simulink model "SS5"  (R2020a)
settings: Solver=VariableStepAuto  StartTime=0.0  StopTime=10.0  RelTol=1e-3
settings Model: Creator=Asus  LastModifiedBy=Asus

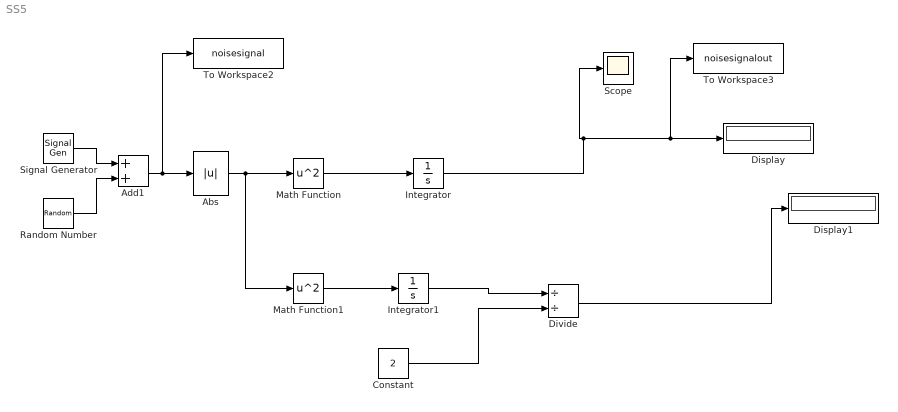
== system SS5 ==
  Abs : Abs
  Add1 : Sum
  Constant : Constant  Value=2
  Display : Display
  Display1 : Display
  Divide : Product  Inputs=//
  Integrator : Integrator  LimitOutput=on
  Integrator1 : Integrator  LimitOutput=on
  Math Function : Math  Operator=square  SaturateOnIntegerOverflow=on
  Math Function1 : Math  Operator=square  SaturateOnIntegerOverflow=on
  Random Number : RandomNumber  SampleTime=0.1
  Scope : Scope
  Signal Generator : SignalGenerator  Units=rad/sec
  To Workspace2 : ToWorkspace  VariableName=noisesignal  SaveFormat=Timeseries  SampleTime=-1
  To Workspace3 : ToWorkspace  VariableName=noisesignalout  SaveFormat=Timeseries  SampleTime=-1
  wires:
  Abs/1 -> Math Function1/1, Math Function/1
  Integrator1/1 -> Divide/1
  Divide/1 -> Display1/1
  Math Function/1 -> Integrator/1
  Math Function1/1 -> Integrator1/1
  Constant/1 -> Divide/2
  Integrator/1 -> To Workspace3/1, Display/1, Scope/1
  Random Number/1 -> Add1/2
  Signal Generator/1 -> Add1/1
  Add1/1 -> To Workspace2/1, Abs/1
